simulink model "Copy_of_minimal_rcu_full"  (R2014b)
settings: Solver=ode4  SolverMode=SingleTasking  StartTime=0.0  StopTime=t_sim  FixedStep=sample_time_model  RelTol=1e-3
PreLoadFcn:
  | initModell
InitFcn:
  | initModell
undefined symbols (not defined in the file): FILTER_TAU_EXT, FIXED_FILTER_BANDWIDTH, FIXED_FILTER_BANDWIDTH_OBSERVER, iter, K_INV, KI2TAU_VEC, KS_trq, KT_trq, load_inertia, load_mass, MAX_CURRENT, MIN_SING_VALUE_M_CART, q0, rCEE_i, sample_time_model, sample_time_robot, tau_max
libraries: simulink x69, robotics x15, beasty_sfcns x7, lwr_dynamics x6, trafo3dLib x4, holgersRobLib x3, dspmtrx3 x1, dspinverses x1
(part 2 of 4)

== system Copy_of_minimal_rcu_full/Roboter+controller/controller/Cartesian Impedance Control/calculate Feedforward ==
  note: Transforming the velocity twist given at the EE in EE coodrinates to impedance point K and K coordnates
  note: get a feedforward term from
      |  the interpolator here
  note: get a switch for interpolator and
      | numerical derivation here
  TCP_T_EE : Inport
  EE_T_K : Inport  Port=2
  0_T_EE_des : Inport  Port=3
  enable Velocity feedforward : Inport  Port=4
  Constant : Constant  Value=0
  Ground : Ground
  Numerische Differentiation : Subsystem
  Product : Product  RndMeth=Zero
  Product1 : Product  Multiplication=Matrix(*)  RndMeth=Zero
  Product2 : Product  Multiplication=Matrix(*)  RndMeth=Zero
  Product3 : Product  Multiplication=Matrix(*)  RndMeth=Zero
  Reshape : Reshape  OutputDimensionality=Customize  OutputDimensions=[4,4]
  Reshape1 : Reshape  OutputDimensionality=Customize  OutputDimensions=[4,4]
  Selector : Selector  NumberOfDimensions=2  InputPortWidth=3  IndexOptions=Index vector (dialog),Index vector (dialog)  Indices=1:3,1:4  OutputSizes=1,1
  Switch : Switch  Criteria=u2 > Threshold
  Trafo3D Adjoint : Subsystem
      mask help: Adjoint matrix for a given frame.
  Trafo3D Inverse : trafo3dLib/Trafo3D Inverse
  check if  matrix  is SO(3) : MATLAB Function  TreatAsAtomicUnit=on
  check if  matrix  is SO(3)1 : MATLAB Function  TreatAsAtomicUnit=on
  prepare matrix : Subsystem
  select 3,1 : Selector  NumberOfDimensions=2  InputPortWidth=3  IndexOptions=Index vector (dialog),Index vector (dialog)  Indices=[1:3],[1:4]  OutputSizes=1,1
  select 3,4 : Selector  NumberOfDimensions=2  InputPortWidth=3  IndexOptions=Index vector (dialog),Index vector (dialog)  Indices=[1:3],[1:4]  OutputSizes=1,1
  TCP_T_k : Outport  OutDataTypeStr=double  PortDimensions=[3 4]
  0_T_K_des : Outport  Port=2  OutDataTypeStr=double  PortDimensions=[3 4]
  dxdes : Outport  Port=3  OutDataTypeStr=double  PortDimensions=[6 1]
  wires:
  select 3,4/1 -> TCP_T_k/1
  select 3,1/1 -> 0_T_K_des/1
  0_T_EE_des/1 -> prepare matrix/1(In1)
  EE_T_K/1 -> Reshape/1
  TCP_T_EE/1 -> Reshape1/1
  Trafo3D Adjoint/1(AdH) -> Product3/1
  Product3/1 -> Product/2
  Switch/1 -> Product3/2
  Numerische Differentiation/1(EE_dx) -> Switch/3
  Product/1 -> dxdes/1
  check if  matrix  is SO(3)/1(EE_T_K) -> Product1/2, Product2/2, Selector/1
  check if  matrix  is SO(3)1/1(TCP_T_EE) -> Product2/1
  Ground/1 -> Switch/1
  Constant/1 -> Switch/2
  Reshape/1 -> check if  matrix  is SO(3)/1(matrix)
  Reshape1/1 -> check if  matrix  is SO(3)1/1(matrix)
  prepare matrix/1(Out1) -> Product1/1, Numerische Differentiation/1(T_des)
  Product2/1 -> select 3,4/1
  Product1/1 -> select 3,1/1
  enable Velocity feedforward/1 -> Product/1
  Selector/1 -> Trafo3D Inverse/1
  Trafo3D Inverse/1 -> Trafo3D Adjoint/1(H)  "K_T_EE"

== system Copy_of_minimal_rcu_full/Roboter+controller/controller/Cartesian Impedance Control/check_settings ==
  In1 : Inport
  Add1 : Sum
  Bus Selector1 : BusSelector  OutputSignals=mEE,rC_EE,I_EE
  Compare To Zero : simulink/Logic and Bit Operations/Compare To Zero  relop===  OutDataTypeStr=uint8  ZeroCross=off
  Compare To Zero1 : simulink/Logic and Bit Operations/Compare To Zero  relop===  OutDataTypeStr=uint8  ZeroCross=off
  Compare To Zero2 : simulink/Logic and Bit Operations/Compare To Zero  relop=<  OutDataTypeStr=uint8  ZeroCross=off
  Compare To Zero3 : simulink/Logic and Bit Operations/Compare To Zero  relop=<  OutDataTypeStr=uint8  ZeroCross=off
  Compare To Zero4 : simulink/Logic and Bit Operations/Compare To Zero  relop=<  OutDataTypeStr=uint8  ZeroCross=off
  Compare To Zero5 : simulink/Logic and Bit Operations/Compare To Zero  relop=~=  OutDataTypeStr=uint8
  Constant1 : Constant  Value=load_mass
  Constant3 : Constant  Value=load_inertia
  Logical Operator : Logic  Operator=OR  Inputs=5  AllPortsSameDT=off  OutDataTypeStr=boolean
  Mux1 : Mux  Inputs=3
  Product : Product  RndMeth=Zero
  Selector : Selector  InputPortWidth=3  Indices=[1]
  Selector1 : Selector  InputPortWidth=3  Indices=[2]
  Selector2 : Selector  InputPortWidth=3  Indices=[3]
  Sum of Elements : Sum  Inputs=+
  Switch : Switch  Criteria=u2 ~= 0
  load_params : Outport
  wires:
  Constant1/1 -> Product/2
  Compare To Zero5/1 -> Product/1
  Product/1 -> Add1/1
  Bus Selector1/2 -> Mux1/2  "<rC_EE>"
  Bus Selector1/3 -> Switch/3, Sum of Elements/1, Selector/1, Selector1/1, Selector2/1  "<I_EE>"
  Bus Selector1/1 -> Compare To Zero/1, Add1/2, Compare To Zero5/1  "<mEE>"
  In1/1 -> Bus Selector1/1
  Mux1/1 -> load_params/1
  Compare To Zero/1 -> Logical Operator/1
  Add1/1 -> Mux1/1
  Constant3/1 -> Switch/1
  Sum of Elements/1 -> Compare To Zero1/1
  Compare To Zero1/1 -> Logical Operator/2
  Compare To Zero2/1 -> Logical Operator/3
  Compare To Zero3/1 -> Logical Operator/4
  Compare To Zero4/1 -> Logical Operator/5
  Selector/1 -> Compare To Zero2/1
  Selector1/1 -> Compare To Zero3/1
  Selector2/1 -> Compare To Zero4/1
  Logical Operator/1 -> Switch/2
  Switch/1 -> Mux1/3

== system Copy_of_minimal_rcu_full/Roboter+controller/controller/Cartesian Impedance Control/easy interpolate ==
  desire : Inport
  rate : Inport  Port=2
  Clock : Clock
  Compare To Constant : simulink/Logic and Bit Operations/Compare To Constant  relop=<=  const=0.001  OutDataTypeStr=uint8  ZeroCross=off
  Logical Operator : Logic  Operator=OR  AllPortsSameDT=off  OutDataTypeStr=boolean
  Relational Operator : RelationalOperator  Operator=~=  OutDataTypeStr=boolean
  Unit Delay : UnitDelay  SampleTime=-1
  easy interpolator inside : Subsystem
  Out : Outport
  wires:
  desire/1 -> easy interpolator inside/1(desire), Relational Operator/2
  rate/1 -> easy interpolator inside/2(rate)
  easy interpolator inside/1(Out) -> Unit Delay/1, Out/1
  Relational Operator/1 -> Logical Operator/1
  Unit Delay/1 -> Relational Operator/1
  Clock/1 -> Compare To Constant/1
  Compare To Constant/1 -> Logical Operator/2
  Logical Operator/1 -> easy interpolator inside/Enable

== system Copy_of_minimal_rcu_full/Roboter+controller/controller/Cartesian Impedance Control/make matrix ==
  In1 : Inport
  Bus Selector1 : BusSelector  OutputSignals=dynamics_q.G,dynamics_q.Mass
  Matrix Concatenation : Concatenate  NumInputs=3  Mode=Multidimensional array  ConcatenateDimension=2
  Reshape1 : Reshape  OutputDimensionality=Customize  OutputDimensions=[7,7]
  zeros : Constant  Value=zeros(7,1)  VectorParams1D=off
  Out1 : Outport
  wires:
  Reshape1/1 -> Matrix Concatenation/3
  Bus Selector1/2 -> Reshape1/1  "<Mass>"
  Bus Selector1/1 -> Matrix Concatenation/1  "<G>"
  In1/1 -> Bus Selector1/1
  Matrix Concatenation/1 -> Out1/1
  zeros/1 -> Matrix Concatenation/2

== system Copy_of_minimal_rcu_full/Roboter+controller/controller/Joint Impedance/JOINT_IMPEDANCE_CONTROL ==
  theta : Inport
  theta_d : Inport  Port=2
  dtheta_d : Inport  Port=3
  ddtheta_d : Inport  Port=4
  enable FFWD_vel : Inport  Port=5
  enable FFWD_acc : Inport  Port=6
  joint_comp_params : Inport  Port=7
  M(theta) : Inport  Port=8
  g(theta) : Inport  Port=9
  dtheta : Inport  Port=10
  B_theta : Inport  Port=11
  Enable : EnablePort
  Joint Compliance Control : Subsystem  TreatAsAtomicUnit=on
  tau_d : Outport
  wires:
  theta/1 -> Joint Compliance Control/2(theta)
  joint_comp_params/1 -> Joint Compliance Control/4(params)
  theta_d/1 -> Joint Compliance Control/1(theta_d)
  M(theta)/1 -> Joint Compliance Control/3(M(theta))
  Joint Compliance Control/1(tau_d) -> tau_d/1
  g(theta)/1 -> Joint Compliance Control/5(g(theta))
  dtheta/1 -> Joint Compliance Control/6(dtheta)
  B_theta/1 -> Joint Compliance Control/7(B_theta)
  dtheta_d/1 -> Joint Compliance Control/8(dtheta_d)
  enable FFWD_vel/1 -> Joint Compliance Control/10(enable FFWD_Vel)
  ddtheta_d/1 -> Joint Compliance Control/9(ddtheta_d)
  enable FFWD_acc/1 -> Joint Compliance Control/11(enable FFWD_Acc)

== system Copy_of_minimal_rcu_full/Roboter+controller/controller/Joint Impedance/Joint Compliance Parameters ==
  K_theta : Inport
  D_theta : Inport  Port=2
  Iterations : Constant  Value=5  OutDataTypeStr=double
  Manual Switch : ManualSwitch
  Mux1 : Mux  Inputs=5
  NO stiffness correction : Constant  Value=0  OutDataTypeStr=double
  Saturation : Saturate  UpperLimit=[2000 2000 2000 2000 2000 800 2000]  LowerLimit=0.001
  Selector : Selector  InputPortWidth=7
  WITH stiffness correction : Constant  OutDataTypeStr=double
  delay : Constant  Value=0  OutDataTypeStr=double
  interpol1 : Subsystem
  interpol2 : Subsystem
  all : Outport
  wires:
  Mux1/1 -> all/1
  NO stiffness correction/1 -> Manual Switch/1
  WITH stiffness correction/1 -> Manual Switch/2
  Iterations/1 -> Mux1/3
  Manual Switch/1 -> Mux1/4
  delay/1 -> Mux1/5
  K_theta/1 -> interpol1/1(In1)
  Saturation/1 -> Mux1/1
  D_theta/1 -> interpol2/1(In1)
  Selector/1 -> Mux1/2
  interpol1/1(Out1) -> Saturation/1
  interpol2/1(Out1) -> Selector/1

== system Copy_of_minimal_rcu_full/Roboter+controller/controller/Joint Impedance/Velocity Filter ==
  q : Inport
  Discrete Filter1 : Subsystem
  Subsystem : Subsystem
  dq : Outport
  wires:
  Discrete Filter1/1(dq_filt) -> dq/1
  q/1 -> Subsystem/1(u), Subsystem/2(y_init)
  Subsystem/1(y) -> Discrete Filter1/1(dq)

== system Copy_of_minimal_rcu_full/Roboter+controller/controller/gains_selector/K_imp ==
  KS_imp : Constant  Value=KS_trq.*[1 1 1 1 1 1 1]*1.0
  KT_imp : Constant  Value=KT_trq.*[1 1 1 1 1 1 1].*[0.8 0.8 0.7 0.8 0.8 0.8 0.8]
  Mux2 : Mux  Inputs=2
  Reshape : Reshape
  K_T : Outport
  K : Outport  Port=2
  wires:
  Mux2/1 -> Reshape/1  "K_imp"
  KS_imp/1 -> Mux2/1
  KT_imp/1 -> Mux2/2, K_T/1  "KT_imp"
  Reshape/1 -> K/1

== system Copy_of_minimal_rcu_full/Roboter+controller/controller/gains_selector/K_imp_joint ==
  KS_imp_joint : Constant  Value=KS_trq.*[1 1 1 1 1 1 1]*1.2
  KT_imp_joint : Constant  Value=KT_trq.*[1 1 1 1 1 1 1].*[1 1 1.2 1 1 1 1]
  Mux4 : Mux  Inputs=2
  Reshape : Reshape
  K_T : Outport
  K : Outport  Port=2
  wires:
  KS_imp_joint/1 -> Mux4/1
  Mux4/1 -> Reshape/1
  Reshape/1 -> K/1
  KT_imp_joint/1 -> Mux4/2, K_T/1  "KT_imp_joint"

== system Copy_of_minimal_rcu_full/Roboter+controller/robot_simulation/Dynamics/Joint Dynamic ==
  note: Calculates the elastic joints from
      | BJoint*d^2theta/dt^2 +KJoint(theta-q)+DJoint/KJoint*(dtheta/dt-dq/dt)+DvisJoint*dtheta/dt = tau_m
      |
      | STANDARD PARAMETERS
      | KJoint = [6900 10854.7 10000 10000 6464.3 10000 10000]
      | BJoint = [4.155 4.155 3.616 1.385 0.541 0.60083 0.60083]
      | DvisJoint = [20 16.98 16.6 24 18 12 12]
      | DJoint = [0 0 0 0 0 0 0]
      | TauMaxJoint = [180 180 80 80 30 30 30]
      |
      | INPUTS
      |    q joint angles
      |    dq/dt joint velocities
      |    tau_m motor torque
      |
      | OUTPUTS
      |    tau_a to the robot applied torque
      |    theta motor position
      |    dtheta/dt motor velocity
  q : Inport
  qd : Inport  Port=2
  tau_m : Inport  Port=3
  tehta_0 : Inport  Port=4
  1/ Bjoint : Gain  Gain=1./[4.155 4.155 3.616 1.385 0.541 0.60083 0.60083]'
  Display2 : Display
  DvisJoint : Gain  Gain=[20 16.98 16.6 24 18 12 12]'
  Integrator1 : Integrator  InitialCondition=zeros(7,1)
  Integrator2 : Integrator  InitialConditionSource=external  InitialCondition=[0; pi/4; 0; pi/4; 0; pi/4; 0]
  Sum : Sum  Inputs=|-+
  Sum1 : Sum  Inputs=|-+
  Sum2 : Sum  Inputs=-+-
  Sum3 : Sum  Inputs=|++
  dJoiunt/kJoint : Gain  Gain=zeros(7,1)
  kJoint : Gain  Gain=[6900 10854.7 10000 10000 6464.3 10000 10000]'
  kJoint1 : Gain  Gain=[6900 10854.7 10000 10000 6464.3 10000 10000]'
  tauMaxJoint : Saturate  UpperLimit=tau_max  LowerLimit=-tau_max
  tau_a : Outport
  theta : Outport  Port=2
  thetaD : Outport  Port=3
  wires:
  kJoint/1 -> dJoiunt/kJoint/1
  tauMaxJoint/1 -> tau_a/1, Sum2/1
  Sum3/1 -> tauMaxJoint/1
  1/ Bjoint/1 -> Integrator1/1
  DvisJoint/1 -> Sum2/3
  kJoint1/1 -> Sum3/2
  Sum1/1 -> kJoint/1
  Sum/1 -> kJoint1/1
  tau_m/1 -> Sum2/2
  Sum2/1 -> 1/ Bjoint/1
  qd/1 -> Sum1/1
  Integrator2/1 -> Display2/1, theta/1, Sum/2  "theta"
  q/1 -> Sum/1
  Integrator1/1 -> thetaD/1, DvisJoint/1, Integrator2/1, Sum1/2  "thetaD"
  dJoiunt/kJoint/1 -> Sum3/1
  tehta_0/1 -> Integrator2/2

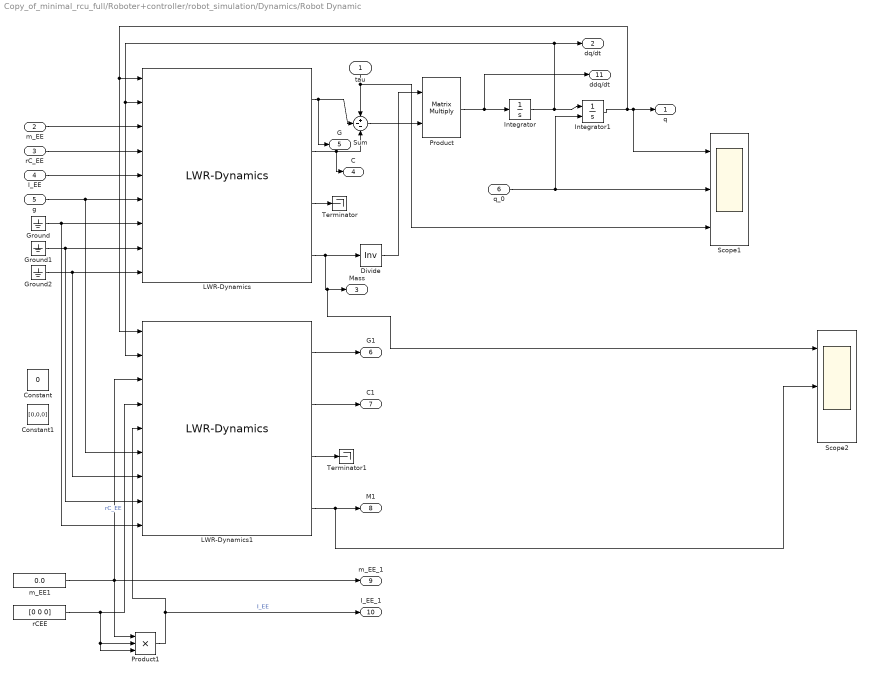
== system Copy_of_minimal_rcu_full/Roboter+controller/robot_simulation/Dynamics/Robot Dynamic ==
  tau : Inport
  m_EE : Inport  Port=2
  rC_EE : Inport  Port=3
  I_EE : Inport  Port=4
  g : Inport  Port=5
  q_0 : Inport  Port=6
  Constant : Constant  Value=0
  Constant1 : Constant  Value=[0,0,0]
  Divide : Product  Inputs=/  Multiplication=Matrix(*)
  Ground : Ground
  Ground1 : Ground
  Ground2 : Ground
  Integrator : Integrator  InitialCondition=zeros(7,1)
  Integrator1 : Integrator  InitialConditionSource=external
  LWR-Dynamics : lwr_dynamics/Dynamics/LWR-Dynamics
  LWR-Dynamics1 : lwr_dynamics/Dynamics/LWR-Dynamics
  Product : Product  Multiplication=Matrix(*)  RndMeth=Zero
  Product1 : Product  Inputs=3  RndMeth=Zero
  Scope1 : Scope  NumInputPorts=3
      settings: TimeRange=2  YMin=-2~-2~-40  YMax=1~1~20
  Scope2 : Scope  NumInputPorts=3
      settings: TimeRange=2  YMin=-0.1~-1~-0.00015  YMax=0.6~1~0.0001  SaveName=ScopeData11
  Sum : Sum  Inputs=+--
  Terminator : Terminator
  Terminator1 : Terminator
  m_EE1 : Constant  Value=0.0
  rCEE : Constant  Value=[0 0 0]
  q : Outport
  dq/dt : Outport  Port=2
  Mass : Outport  Port=3
  C : Outport  Port=4
  G : Outport  Port=5
  G1 : Outport  Port=6
  C1 : Outport  Port=7
  M1 : Outport  Port=8
  m_EE_1 : Outport  Port=9
  I_EE_1 : Outport  Port=10
  ddq/dt : Outport  Port=11
  wires:
  Integrator/1 -> Integrator1/1, dq/dt/1, LWR-Dynamics1/2, LWR-Dynamics/2
  LWR-Dynamics/4 -> Divide/1, Scope2/1, Mass/1
  LWR-Dynamics/1 -> Sum/2, G/1
  Sum/1 -> Product/2
  Integrator1/1 -> Scope1/1, q/1, LWR-Dynamics1/1, LWR-Dynamics/1
  m_EE/1 -> LWR-Dynamics/3
  rC_EE/1 -> LWR-Dynamics/4
  I_EE/1 -> LWR-Dynamics/5
  Ground/1 -> LWR-Dynamics1/9, LWR-Dynamics/7
  Ground1/1 -> LWR-Dynamics/8, LWR-Dynamics1/8
  Ground2/1 -> LWR-Dynamics/9, LWR-Dynamics1/7
  Divide/1 -> Product/1
  Product/1 -> ddq/dt/1, Integrator/1
  g/1 -> LWR-Dynamics/6, LWR-Dynamics1/6
  LWR-Dynamics/2 -> Sum/3, C/1
  tau/1 -> Sum/1, Scope1/3
  LWR-Dynamics/3 -> Terminator/1
  q_0/1 -> Integrator1/2, Scope1/2
  LWR-Dynamics1/3 -> Terminator1/1
  LWR-Dynamics1/1 -> G1/1
  LWR-Dynamics1/2 -> C1/1
  LWR-Dynamics1/4 -> Scope2/2, M1/1
  rCEE/1 -> LWR-Dynamics1/4, Product1/2, Product1/3  "rC_EE"
  m_EE1/1 -> LWR-Dynamics1/3, m_EE_1/1, Product1/1
  Product1/1 -> LWR-Dynamics1/5, I_EE_1/1  "I_EE"

== system Copy_of_minimal_rcu_full/Roboter+controller/robot_simulation/Dynamics/ZUSTANDSREGLER1 ==
  note: tau_m
  tau : Inport
  tau_d : Inport  Port=2
  Gains : Inport  Port=3
  dCG_0 : Inport  Port=4
  reset : Inport  Port=5
  CG_0 : Inport  Port=6
  Joint_controller joint_impedance : Subsystem
  Saturation : Saturate  UpperLimit=MAX_CURRENT  LowerLimit=-MAX_CURRENT
  Selctor : Selector  InputPortWidth=14  Indices=1:7
  Selctor1 : Selector  InputPortWidth=14  Indices=8:14
  Sum : Sum  Inputs=++|
  Sum1 : Sum  Inputs=|++
  Torque comp1 : Gain  Gain=KI2TAU_VEC  SaturateOnIntegerOverflow=on  OutDataTypeStr=Inherit: Same as input  ParamDataTypeStr=Inherit: Same as input
  controller cart impedance : Subsystem
  Current_des : Outport  InitialOutput=0
  wires:
  tau_d/1 -> Sum/1, Joint_controller joint_impedance/1(tau_d), controller cart impedance/1(tau_d)  "tau_d"
  Torque comp1/1 -> Saturation/1
  Saturation/1 -> Current_des/1
  CG_0/1 -> controller cart impedance/2(CG_0), Joint_controller joint_impedance/2(CG_O)  "CG_O"
  Joint_controller joint_impedance/1(I_out) -> Sum1/2
  controller cart impedance/1(I_out) -> Sum1/1
  Sum/1 -> Torque comp1/1
  reset/1 -> Joint_controller joint_impedance/5(reset), controller cart impedance/5(reset)
  Sum1/1 -> Sum/2
  Gains/1 -> Selctor/1, Selctor1/1
  dCG_0/1 -> controller cart impedance/6(dCG_0)
  tau/1 -> controller cart impedance/3(tau), Joint_controller joint_impedance/3(tau)  "tau"
  Selctor/1 -> controller cart impedance/4(Gains)
  Selctor1/1 -> Joint_controller joint_impedance/4(Gains)

== system Copy_of_minimal_rcu_full/Roboter+controller/robot_simulation/model/Body Jacobians ==
  q : Inport
  TCP_T_EE : Inport  Port=2
  Bus Creator1 : BusCreator  Inputs=8
  Jacobian LBR-M : S-Function  FunctionName=lbrmjacobitcp_sfun  EnableBusSupport=off
  Math Function : Math  Operator=transpose  SaturateOnIntegerOverflow=on
  Reshape{,1..7} (8 alike) : Reshape
  Reshape8 : Reshape  OutputDimensionality=Customize  OutputDimensions=[4,4]
  S-Function : S-Function  FunctionName=KUKA_JacobianTotTransposedSfun  Parameters=rot(1,1), rot(1,2), rot(1,3), rot(2,1), rot(2,2), rot(2,3), rot(3,1), rot(3,2), rot(3,3), tcp(1), tcp(2), tcp(3)  EnableBusSupport=off  mask{rot=eye(3), tcp=zeros(3,1)}
      mask prompts: rot "TCP-Rotation"; tcp "TCP-Translation"
  Selector : Selector  NumberOfDimensions=2  InputPortWidth=3  IndexOptions=Select all,Index vector (dialog)  Indices=-1,1:6
  Selector1 : Selector  NumberOfDimensions=2  InputPortWidth=3  IndexOptions=Select all,Index vector (dialog)  Indices=-1,7:12
  Selector2 : Selector  NumberOfDimensions=2  InputPortWidth=3  IndexOptions=Select all,Index vector (dialog)  Indices=-1,13:18
  Selector3 : Selector  NumberOfDimensions=2  InputPortWidth=3  IndexOptions=Select all,Index vector (dialog)  Indices=-1,19:24
  Selector4 : Selector  NumberOfDimensions=2  InputPortWidth=3  IndexOptions=Select all,Index vector (dialog)  Indices=-1,25:30
  Selector5 : Selector  NumberOfDimensions=2  InputPortWidth=3  IndexOptions=Select all,Index vector (dialog)  Indices=-1,31:36
  Selector6 : Selector  NumberOfDimensions=2  InputPortWidth=3  IndexOptions=Select all,Index vector (dialog)  Indices=-1,37:42
  Selector7 : Selector  NumberOfDimensions=2  InputPortWidth=3  IndexOptions=Index vector (dialog),Index vector (dialog)  Indices=1:3,1:4
  jacobians wrt body : Outport
  wires:
  Math Function/1 -> Reshape7/1
  Selector7/1 -> Jacobian LBR-M/2
  Reshape8/1 -> Selector7/1
  Reshape7/1 -> Bus Creator1/8  "B_JT_EE"
  Jacobian LBR-M/1 -> Math Function/1
  TCP_T_EE/1 -> Reshape8/1
  Bus Creator1/1 -> jacobians wrt body/1
  Reshape6/1 -> Bus Creator1/7  "B_JT_7"
  Reshape5/1 -> Bus Creator1/6  "B_JT_6"
  Reshape4/1 -> Bus Creator1/5  "B_JT_5"
  Reshape3/1 -> Bus Creator1/4  "B_JT_4"
  Reshape2/1 -> Bus Creator1/3  "B_JT_3"
  Reshape1/1 -> Bus Creator1/2  "B_JT_2"
  Reshape/1 -> Bus Creator1/1  "B_JT_1"
  q/1 -> Jacobian LBR-M/1, S-Function/1
  Selector/1 -> Reshape/1
  Selector1/1 -> Reshape1/1
  Selector2/1 -> Reshape2/1
  Selector3/1 -> Reshape3/1
  Selector4/1 -> Reshape4/1
  Selector5/1 -> Reshape5/1
  Selector6/1 -> Reshape6/1
  S-Function/1 -> Selector/1, Selector1/1, Selector2/1, Selector3/1, Selector4/1, Selector6/1, Selector5/1

== system Copy_of_minimal_rcu_full/Roboter+controller/robot_simulation/model/Jacobians to Zero ==
  q : Inport
  TCP_T_EE : Inport  Port=2
  Bus Creator1 : BusCreator  Inputs=8
  LWR Jacobian EE : lwr_dynamics/Kinematics/LWR Jacobian EE
  LWR-Jacobians : lwr_dynamics/Kinematics/LWR-Jacobians
  Reshape{1..8} (8 alike) : Reshape
  Reshape9 : Reshape  OutputDimensionality=Customize  OutputDimensions=[4,4]
  jacobians_wrt_zero : Outport
  wires:
  Reshape9/1 -> LWR Jacobian EE/2
  Reshape8/1 -> Bus Creator1/8  "O_JT_EE"
  Reshape7/1 -> Bus Creator1/7  "O_JT_7"
  Reshape6/1 -> Bus Creator1/6  "O_JT_6"
  Reshape5/1 -> Bus Creator1/5  "O_JT_5"
  Reshape3/1 -> Bus Creator1/4  "O_JT_4"
  Reshape2/1 -> Bus Creator1/3  "O_JT_3"
  Reshape1/1 -> Bus Creator1/2  "O_JT_2"
  Reshape4/1 -> Bus Creator1/1  "O_JT_1"
  q/1 -> LWR-Jacobians/1, LWR Jacobian EE/1
  LWR Jacobian EE/1 -> Reshape8/1
  LWR-Jacobians/7 -> Reshape7/1
  LWR-Jacobians/6 -> Reshape6/1
  LWR-Jacobians/5 -> Reshape5/1
  LWR-Jacobians/4 -> Reshape3/1
  LWR-Jacobians/3 -> Reshape2/1
  LWR-Jacobians/2 -> Reshape1/1
  LWR-Jacobians/1 -> Reshape4/1
  TCP_T_EE/1 -> Reshape9/1
  Bus Creator1/1 -> jacobians_wrt_zero/1

== system Copy_of_minimal_rcu_full/Roboter+controller/robot_simulation/model/forward_kin_q ==
  q : Inport
  TCP_T_EE : Inport  Port=2
  Bus Creator2 : BusCreator  Inputs=9
  Gain : Gain
  LWR-Transformations : lwr_dynamics/Kinematics/LWR-Transformations
  fkin_q : Outport
  wires:
  LWR-Transformations/8 -> Bus Creator2/9  "O_T_EE"
  Bus Creator2/1 -> fkin_q/1
  Gain/1 -> Bus Creator2/8  "O_T_TCP"
  LWR-Transformations/7 -> Bus Creator2/7, Gain/1  "O_T_7"
  LWR-Transformations/6 -> Bus Creator2/6  "O_T_6"
  LWR-Transformations/5 -> Bus Creator2/5  "O_T_5"
  LWR-Transformations/4 -> Bus Creator2/4  "O_T_4"
  LWR-Transformations/3 -> Bus Creator2/3  "O_T_3"
  LWR-Transformations/2 -> Bus Creator2/2  "O_T_2"
  LWR-Transformations/1 -> Bus Creator2/1  "O_T_1"
  q/1 -> LWR-Transformations/1
  TCP_T_EE/1 -> LWR-Transformations/2

== system Copy_of_minimal_rcu_full/Roboter+controller/robot_simulation/model/forward_kin_q1 ==
  q : Inport
  TCP_T_EE : Inport  Port=2
  Bus Creator2 : BusCreator  Inputs=9
  Gain : Gain
  LWR-Transformations : lwr_dynamics/Kinematics/LWR-Transformations
  fkin_q : Outport
  wires:
  TCP_T_EE/1 -> LWR-Transformations/2
  q/1 -> LWR-Transformations/1
  LWR-Transformations/1 -> Bus Creator2/1  "O_T_1"
  LWR-Transformations/2 -> Bus Creator2/2  "O_T_2"
  LWR-Transformations/3 -> Bus Creator2/3  "O_T_3"
  LWR-Transformations/4 -> Bus Creator2/4  "O_T_4"
  LWR-Transformations/5 -> Bus Creator2/5  "O_T_5"
  LWR-Transformations/6 -> Bus Creator2/6  "O_T_6"
  LWR-Transformations/7 -> Gain/1, Bus Creator2/7  "O_T_7"
  Gain/1 -> Bus Creator2/8  "O_T_TCP"
  Bus Creator2/1 -> fkin_q/1
  LWR-Transformations/8 -> Bus Creator2/9  "O_T_EE"

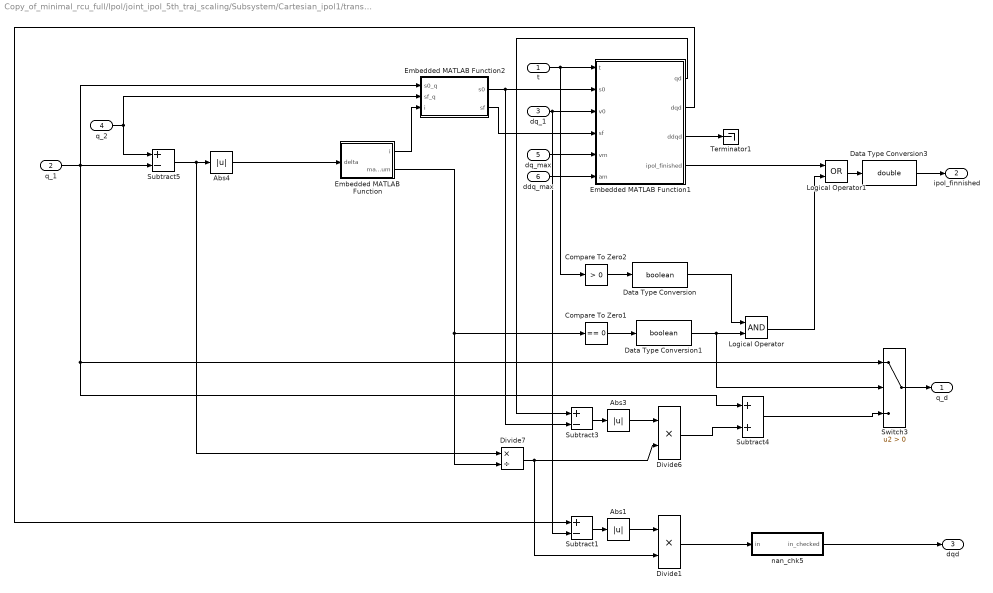
== system Copy_of_minimal_rcu_full/Ipol/joint_ipol_5th_traj_scaling/Subsystem/Cartesian_ipol1/translation ==
  t : Inport
  q_1 : Inport  Port=2
  dq_1 : Inport  Port=3
  q_2 : Inport  Port=4
  dq_max : Inport  Port=5
  ddq_max : Inport  Port=6
  Abs1 : Abs
  Abs3 : Abs
  Abs4 : Abs
  Compare To Zero1 : simulink/Logic and Bit Operations/Compare To Zero  relop===  OutDataTypeStr=uint8  ZeroCross=off
  Compare To Zero2 : simulink/Logic and Bit Operations/Compare To Zero  relop=>  OutDataTypeStr=uint8  ZeroCross=off
  Data Type Conversion : DataTypeConversion  OutDataTypeStr=boolean
  Data Type Conversion1 : DataTypeConversion  OutDataTypeStr=boolean
  Data Type Conversion3 : DataTypeConversion  OutDataTypeStr=double
  Divide1 : Product  Inputs=**
  Divide6 : Product  Inputs=**
  Divide7 : Product  Inputs=*/
  Embedded MATLAB Function : MATLAB Function  TreatAsAtomicUnit=on
  Embedded MATLAB Function1 : MATLAB Function  TreatAsAtomicUnit=on
  Embedded MATLAB Function2 : MATLAB Function  TreatAsAtomicUnit=on
  Logical Operator : Logic  AllPortsSameDT=off  OutDataTypeStr=boolean
  Logical Operator1 : Logic  Operator=OR  AllPortsSameDT=off  OutDataTypeStr=boolean
  Subtract1 : Sum  Inputs=+-
  Subtract3 : Sum  Inputs=+-
  Subtract4 : Sum
  Subtract5 : Sum  Inputs=+-
  Switch3 : Switch  Criteria=u2 > Threshold
  Terminator1 : Terminator
  nan_chk5 : Subsystem
  q_d : Outport
  ipol_finnished : Outport  Port=2
  dqd : Outport  Port=3
  wires:
  nan_chk5/1(in_checked) -> dqd/1
  Divide1/1 -> nan_chk5/1(in)
  Embedded MATLAB Function1/2(dqd) -> Subtract1/1
  Subtract1/1 -> Abs1/1
  Abs1/1 -> Divide1/1
  Divide6/1 -> Subtract4/2
  Divide7/1 -> Divide1/2, Divide6/2
  Abs4/1 -> Embedded MATLAB Function/1(delta)
  Subtract5/1 -> Divide7/1, Abs4/1
  q_1/1 -> Switch3/1, Subtract4/1, Subtract5/2, Embedded MATLAB Function2/1(s0_q)
  q_2/1 -> Subtract5/1, Embedded MATLAB Function2/2(sf_q)
  Embedded MATLAB Function/2(maximum) -> Compare To Zero1/1, Divide7/2
  Embedded MATLAB Function/1(i) -> Embedded MATLAB Function2/3(i)
  Subtract3/1 -> Abs3/1
  dq_1/1 -> Subtract1/2, Embedded MATLAB Function1/3(v0)
  dq_max/1 -> Embedded MATLAB Function1/5(vm)
  ddq_max/1 -> Embedded MATLAB Function1/6(am)
  t/1 -> Embedded MATLAB Function1/1(t), Compare To Zero2/1
  Embedded MATLAB Function2/1(s0) -> Embedded MATLAB Function1/2(s0), Subtract3/2
  Embedded MATLAB Function2/2(sf) -> Embedded MATLAB Function1/4(sf)
  Embedded MATLAB Function1/1(qd) -> Subtract3/1
  Embedded MATLAB Function1/3(ddqd) -> Terminator1/1
  Abs3/1 -> Divide6/1
  Logical Operator/1 -> Logical Operator1/2
  Data Type Conversion/1 -> Logical Operator/1
  Data Type Conversion1/1 -> Logical Operator/2, Switch3/2
  Compare To Zero1/1 -> Data Type Conversion1/1
  Embedded MATLAB Function1/4(ipol_finished) -> Logical Operator1/1
  Logical Operator1/1 -> Data Type Conversion3/1
  Data Type Conversion3/1 -> ipol_finnished/1
  Subtract4/1 -> Switch3/3
  Switch3/1 -> q_d/1
  Compare To Zero2/1 -> Data Type Conversion/1

== system Copy_of_minimal_rcu_full/Ipol/joint_ipol_5th_traj_scaling/Subsystem/time_generator and resets/Triggered Subsystem ==
  t : Inport
  Trigger : TriggerPort
  t0 : Outport
  wires:
  t/1 -> t0/1

== system Copy_of_minimal_rcu_full/Roboter+controller/State_Observer/Impulse_Observer/Subsystem1/calc_beta ==
  M : Inport
  dq : Inport  Port=2
  n : Inport  Port=3
  Discrete Derivative : simulink/Discrete/Discrete Derivative  gainval=1.0  ICPrevScaledInput=0.0  InputProcessing=Inherited  OutMin=[]  OutMax=[]  OutDataType=sfix(16)  OutScaling=2^-10  DoSatur=off
  Product : Product  Multiplication=Matrix(*)  RndMeth=Zero
  Reshape1 : Reshape  OutputDimensionality=Column vector (2-D)
  Reshape2 : Reshape
  Sum6 : Sum  Inputs=+-
  "beta " : Outport
  dM : Outport  Port=2
  dMdq2 : Outport  Port=3
  wires:
  Product/1 -> Reshape2/1
  Discrete Derivative/1 -> dM/1, Product/1
  Sum6/1 -> "beta "/1
  n/1 -> Sum6/1
  M/1 -> Discrete Derivative/1
  dq/1 -> Reshape1/1
  Reshape1/1 -> Product/2
  Reshape2/1 -> dMdq2/1, Sum6/2

== system Copy_of_minimal_rcu_full/Roboter+controller/State_Observer/Impulse_Observer/Subsystem1/calc_p ==
  M : Inport
  dq : Inport  Port=2
  Product : Product  Multiplication=Matrix(*)  RndMeth=Zero
  Reshape : Reshape  OutputDimensionality=Column vector (2-D)
  p : Outport
  wires:
  dq/1 -> Reshape/1
  M/1 -> Product/1
  Product/1 -> p/1
  Reshape/1 -> Product/2

== system Copy_of_minimal_rcu_full/Roboter+controller/controller/Cartesian Impedance Control/Cartesian Compliance Parameters1/damping type ==
  Controller type : Constant  Value=damping_type  OutDataTypeStr=double
  Out1 : Outport
  wires:
  Controller type/1 -> Out1/1

== system Copy_of_minimal_rcu_full/Roboter+controller/controller/Cartesian Impedance Control/Cartesian Compliance Parameters1/interpol ==
  In1 : Inport
  Easy Ipol_MIMO : beasty_sfcns/Utility Functions/Easy Ipol_MIMO  h=sample_time_robot  n=6
  K rates : Constant  Value=[2000 2000 2000 600 600 600]
  Out1 : Outport
  wires:
  In1/1 -> Easy Ipol_MIMO/1
  Easy Ipol_MIMO/1 -> Out1/1  "K_x"
  K rates/1 -> Easy Ipol_MIMO/2, Easy Ipol_MIMO/3

== system Copy_of_minimal_rcu_full/Roboter+controller/controller/Cartesian Impedance Control/Cartesian Compliance Parameters1/interpol5 ==
  In1 : Inport
  Easy Ipol_MIMO : beasty_sfcns/Utility Functions/Easy Ipol_MIMO  h=sample_time_robot  n=6
  K rates3 : Constant  Value=[1 1 1 1 1 1]
  Out1 : Outport
  wires:
  K rates3/1 -> Easy Ipol_MIMO/2, Easy Ipol_MIMO/3
  In1/1 -> Easy Ipol_MIMO/1
  Easy Ipol_MIMO/1 -> Out1/1

== system Copy_of_minimal_rcu_full/Roboter+controller/controller/Cartesian Impedance Control/Cartesian Compliance Parameters1/stiffness type ==
  Controller type : Constant  Value=controller_type  OutDataTypeStr=double
  Out1 : Outport
  wires:
  Controller type/1 -> Out1/1

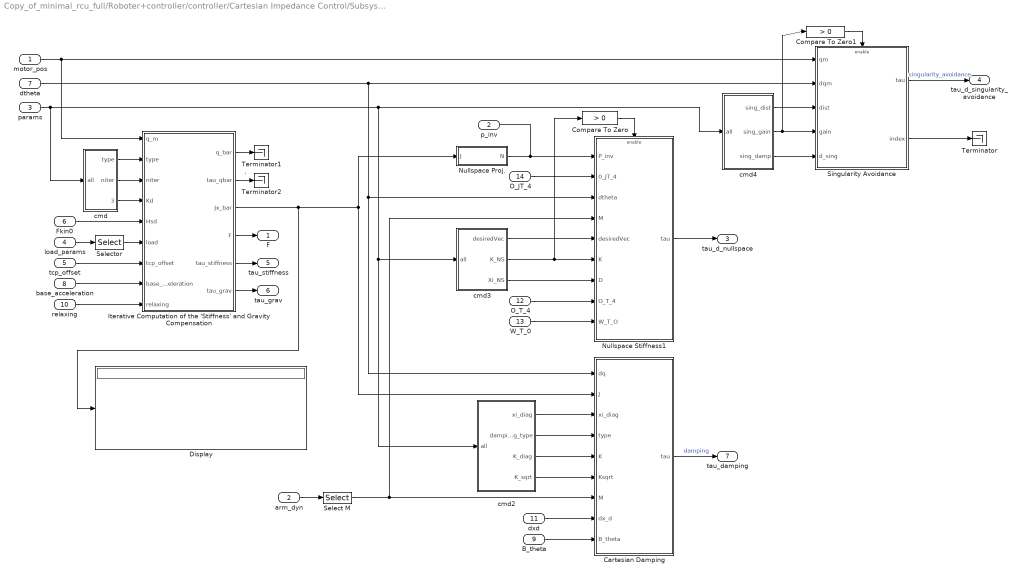
== system Copy_of_minimal_rcu_full/Roboter+controller/controller/Cartesian Impedance Control/Subsystem/Cartesian Compliance Control ==
  motor_pos : Inport
  arm_dyn : Inport  Port=2
  params : Inport  Port=3
  load_params : Inport  Port=4
  tcp_offset : Inport  Port=5
  Fkin0 : Inport  Port=6
  dtheta : Inport  Port=7
  base_acceleration : Inport  Port=8
  B_theta : Inport  Port=9
  relaxing : Inport  Port=10
  dxd : Inport  Port=11
  O_T_4 : Inport  Port=12
  W_T_0 : Inport  Port=13
  O_JT_4 : Inport  Port=14
  Cartesian Damping : Subsystem  TreatAsAtomicUnit=on
  Compare To Zero : simulink/Logic and Bit Operations/Compare To Zero  relop=>  OutDataTypeStr=uint8  ZeroCross=off
  Compare To Zero1 : simulink/Logic and Bit Operations/Compare To Zero  relop=>  OutDataTypeStr=uint8  ZeroCross=off
  Display : Display
  Iterative Computation of the 'Stiffness' and Gravity Compensation : Subsystem  TreatAsAtomicUnit=on
  Nullspace Proj. : MATLAB Function  TreatAsAtomicUnit=on
  Nullspace Stiffness1 : Subsystem  TreatAsAtomicUnit=on
  Select M : Selector  NumberOfDimensions=2  InputPortWidth=3  IndexOptions=Select all,Index vector (dialog)  Indices=-1,3:9
  Selector : Selector  InputPortWidth=7  Indices=1:4
  Singularity Avoidance : Subsystem  TreatAsAtomicUnit=on
  Terminator : Terminator
  Terminator1 : Terminator
  Terminator2 : Terminator
  cmd : Subsystem
  cmd2 : Subsystem
  cmd3 : Subsystem
  cmd4 : Subsystem
  F : Outport  OutDataTypeStr=double  PortDimensions=6
  p_inv : Outport  Port=2  OutDataTypeStr=double  PortDimensions=[7 7]
  tau_d_nullspace : Outport  Port=3  OutDataTypeStr=double  PortDimensions=7
  tau_d_singularity_avoidance : Outport  Port=4  OutDataTypeStr=double  PortDimensions=7
  tau_stiffness : Outport  Port=5  OutDataTypeStr=double  PortDimensions=7
  tau_grav : Outport  Port=6  OutDataTypeStr=double  PortDimensions=7
  tau_damping : Outport  Port=7  OutDataTypeStr=double  PortDimensions=7
  wires:
  base_acceleration/1 -> Iterative Computation of the 'Stiffness' and Gravity Compensation/8(base_acceleration)
  load_params/1 -> Selector/1
  arm_dyn/1 -> Select M/1
  params/1 -> cmd/1(all), cmd2/1(all), cmd3/1(all), cmd4/1(all)
  Singularity Avoidance/1(tau) -> tau_d_singularity_avoidance/1  "singularity_avoidance"
  Compare To Zero/1 -> Nullspace Stiffness1/Enable
  Compare To Zero1/1 -> Singularity Avoidance/Enable
  Cartesian Damping/1(tau) -> tau_damping/1  "damping"
  cmd/3(K_diag) -> Iterative Computation of the 'Stiffness' and Gravity Compensation/4(Kd)
  Iterative Computation of the 'Stiffness' and Gravity Compensation/3(Jx_bar) -> Display/1, Nullspace Proj./1(J), Cartesian Damping/2(J)
  cmd/2(niter) -> Iterative Computation of the 'Stiffness' and Gravity Compensation/3(niter)
  Selector/1 -> Iterative Computation of the 'Stiffness' and Gravity Compensation/6(load)
  cmd/1(type) -> Iterative Computation of the 'Stiffness' and Gravity Compensation/2(type)
  Fkin0/1 -> Iterative Computation of the 'Stiffness' and Gravity Compensation/5(Hsd)
  Iterative Computation of the 'Stiffness' and Gravity Compensation/4(F) -> F/1
  tcp_offset/1 -> Iterative Computation of the 'Stiffness' and Gravity Compensation/7(tcp_offset)
  motor_pos/1 -> Singularity Avoidance/1(qm), Iterative Computation of the 'Stiffness' and Gravity Compensation/1(q_m)
  B_theta/1 -> Cartesian Damping/9(B_theta)
  relaxing/1 -> Iterative Computation of the 'Stiffness' and Gravity Compensation/9(relaxing)
  dxd/1 -> Cartesian Damping/8(dx_d)
  Nullspace Stiffness1/1(tau) -> tau_d_nullspace/1
  O_T_4/1 -> Nullspace Stiffness1/8(O_T_4)
  W_T_0/1 -> Nullspace Stiffness1/9(W_T_O)
  Nullspace Proj./1(N) -> Nullspace Stiffness1/1(P_inv), p_inv/1
  Iterative Computation of the 'Stiffness' and Gravity Compensation/1(q_bar) -> Terminator1/1
  Iterative Computation of the 'Stiffness' and Gravity Compensation/2(tau_qbar) -> Terminator2/1  "'"
  Singularity Avoidance/2(index) -> Terminator/1
  O_JT_4/1 -> Nullspace Stiffness1/2(0_JT_4)
  Select M/1 -> Cartesian Damping/7(M), Nullspace Stiffness1/4(M)
  Iterative Computation of the 'Stiffness' and Gravity Compensation/5(tau_stiffness) -> tau_stiffness/1
  Iterative Computation of the 'Stiffness' and Gravity Compensation/6(tau_grav) -> tau_grav/1
  cmd2/1(xi_diag) -> Cartesian Damping/3(xi_diag)
  cmd2/2(damping_type) -> Cartesian Damping/4(type)
  cmd2/3(K_diag) -> Cartesian Damping/5(K)
  cmd2/4(K_sqrt) -> Cartesian Damping/6(Ksqrt)
  dtheta/1 -> Cartesian Damping/1(dq), Nullspace Stiffness1/3(dtheta), Singularity Avoidance/2(dqm)
  cmd3/1(desiredVec) -> Nullspace Stiffness1/5(desiredVec)
  cmd3/2(K_NS) -> Nullspace Stiffness1/6(K), Compare To Zero/1
  cmd3/3(Xi_NS) -> Nullspace Stiffness1/7(D)
  cmd4/1(sing_dist) -> Singularity Avoidance/3(dist)
  cmd4/2(sing_gain) -> Singularity Avoidance/4(gain), Compare To Zero1/1
  cmd4/3(sing_damp) -> Singularity Avoidance/5(d_sing)

== system Copy_of_minimal_rcu_full/Roboter+controller/controller/Cartesian Impedance Control/Velocity Filter/Discrete Filter1 ==
  dq : Inport
  Add1 : Sum
  Gain1 : Gain  Gain=1/10
  Gain2 : Gain  Gain=9/10
  Unit Delay : UnitDelay  SampleTime=-1
  dq_filt : Outport  OutDataTypeStr=double  PortDimensions=7
  wires:
  dq/1 -> Gain1/1
  Gain1/1 -> Add1/1
  Gain2/1 -> Add1/2
  Add1/1 -> dq_filt/1, Unit Delay/1
  Unit Delay/1 -> Gain2/1

== system Copy_of_minimal_rcu_full/Roboter+controller/controller/Cartesian Impedance Control/calculate Feedforward/Numerische Differentiation ==
  note: Rotate the velocities 0_dx at EE from base coordinates 0 in EE coordinates
  T_des : Inport
  Product2 : Product  Multiplication=Matrix(*)  RndMeth=Zero
  Rotate_wrench1 : Subsystem
      mask help: Adjoint matrix for a given frame.
  Selector : Selector  NumberOfDimensions=2  InputPortWidth=3  IndexOptions=Index vector (dialog),Index vector (dialog)  Indices=1:3,1:4  OutputSizes=1,1
  Trafo3D Inverse : trafo3dLib/Trafo3D Inverse
  nan_chk4 : Subsystem
  numerical differentiation : Subsystem
  EE_dx : Outport
  wires:
  Rotate_wrench1/1(A_R_B) -> nan_chk4/1(in)
  numerical differentiation/1(0_dx) -> Product2/2  "0_dx"
  nan_chk4/1(in_checked) -> Product2/1
  T_des/1 -> numerical differentiation/1(T_des), Selector/1
  Product2/1 -> EE_dx/1
  Trafo3D Inverse/1 -> Rotate_wrench1/1(A_T_B)
  Selector/1 -> Trafo3D Inverse/1

== system Copy_of_minimal_rcu_full/Roboter+controller/controller/Cartesian Impedance Control/calculate Feedforward/Trafo3D Adjoint ==
  H : Inport
  0 : Constant  Value=zeros(3,3)  VectorParams1D=off
  Cross-Product : trafo3dLib/Cross-Product  SystemSampleTime=-1
  Matrix Concatenation : Concatenate  Mode=Multidimensional array  ConcatenateDimension=2
  Matrix Concatenation1 : Concatenate  Mode=Multidimensional array
  Matrix Concatenation2 : Concatenate  Mode=Multidimensional array  ConcatenateDimension=2
  R : Selector  NumberOfDimensions=2  InputPortWidth=3  IndexOptions=Index vector (dialog),Index vector (dialog)  Indices=[1,2,3],[1 2 3]
  p : Selector  NumberOfDimensions=2  InputPortWidth=3  IndexOptions=Index vector (dialog),Index vector (dialog)  Indices=[1 2 3],4
  AdH : Outport
  wires:
  Matrix Concatenation1/1 -> AdH/1
  Matrix Concatenation2/1 -> Matrix Concatenation1/2
  Cross-Product/1 -> Matrix Concatenation/2
  Matrix Concatenation/1 -> Matrix Concatenation1/1
  0/1 -> Matrix Concatenation2/1
  H/1 -> p/1, R/1
  p/1 -> Cross-Product/1
  R/1 -> Cross-Product/2, Matrix Concatenation2/2, Matrix Concatenation/1

== system Copy_of_minimal_rcu_full/Roboter+controller/controller/Cartesian Impedance Control/calculate Feedforward/prepare matrix ==
  In1 : Inport
  Constant1 : Constant  Value=[0 0 0 1]  VectorParams1D=off
  Matrix Concatenate : Concatenate  Mode=Multidimensional array
  Reshape2 : Reshape  OutputDimensionality=Customize  OutputDimensions=[3,4]
  Out1 : Outport
  wires:
  Reshape2/1 -> Matrix Concatenate/1
  Constant1/1 -> Matrix Concatenate/2
  Matrix Concatenate/1 -> Out1/1
  In1/1 -> Reshape2/1

== system Copy_of_minimal_rcu_full/Roboter+controller/controller/Cartesian Impedance Control/easy interpolate/easy interpolator inside ==
  desire : Inport
  rate : Inport  Port=2
  Enable : EnablePort
  Abs : Abs
  Detect Change : simulink/Logic and Bit Operations/Detect Change  vinit=0  InputProcessing=Inherited  OutDataTypeStr=uint8
  Discrete-Time Integrator : DiscreteIntegrator  ExternalReset=rising  InitialConditionSource=external  SampleTime=-1
  Display{1..7} (7 alike) : Display
  MinMax : MinMax  Inputs=2
  MinMax1 : MinMax  Function=max  Inputs=2
  Product : Product  RndMeth=Zero
  Saturation Dynamic : simulink/Discontinuities/Saturation Dynamic  OutMin=[]  OutMax=[]  OutDataTypeStr=Inherit: Same as second input  OutDataType=sfix(16)  OutScaling=2^-10  DoSatur=off
  Unit Delay External IC : simulink/Additional Math & Discrete/Additional Discrete/Unit Delay External IC  tsamp=-1
  correct sign : Subsystem
  memorize last : Subsystem
  Out : Outport
  wires:
  desire/1 -> memorize last/1(In1), correct sign/2(In2), Detect Change/1, MinMax1/1, MinMax/1, Unit Delay External IC/2, Display2/1
  memorize last/1(Out1) -> correct sign/1(In1), MinMax1/2, MinMax/2, Display7/1
  rate/1 -> Abs/1
  correct sign/1(Out1) -> Product/1
  Abs/1 -> Product/2
  Product/1 -> Discrete-Time Integrator/1
  Detect Change/1 -> Discrete-Time Integrator/2
  Discrete-Time Integrator/1 -> Saturation Dynamic/2, Display4/1
  MinMax1/1 -> Display1/1, Saturation Dynamic/1, Display5/1
  MinMax/1 -> Saturation Dynamic/3, Display6/1
  Saturation Dynamic/1 -> Out/1, Unit Delay External IC/1, Display3/1
  Unit Delay External IC/1 -> Discrete-Time Integrator/3

== system Copy_of_minimal_rcu_full/Roboter+controller/controller/Joint Impedance/JOINT_IMPEDANCE_CONTROL/Joint Compliance Control ==
  theta_d : Inport
  theta : Inport  Port=2
  M(theta) : Inport  Port=3
  params : Inport  Port=4
  g(theta) : Inport  Port=5
  dtheta : Inport  Port=6
  B_theta : Inport  Port=7
  dtheta_d : Inport  Port=8
  ddtheta_d : Inport  Port=9
  enable FFWD_Vel : Inport  Port=10
  enable FFWD_Acc : Inport  Port=11
  Add : Sum
  Damping Design via Generalized Eigenvalues : Subsystem
  Embedded MATLAB Function : MATLAB Function  TreatAsAtomicUnit=on
  Multiport Switch1 : MultiPortSwitch  DataPortOrder=Zero-based contiguous  Inputs=6  zeroidx=on
  NAN_checks : Subsystem
  Pragmatic Solution : Subsystem  TreatAsAtomicUnit=on
  Reshape1 : Reshape  OutputDimensionality=Customize  OutputDimensions=[7,7]
  Unit Delay{,1..4} (5 alike) : UnitDelay  SampleTime=sample_time_model
  cmd : Subsystem
  tau_d : Outport
  wires:
  params/1 -> cmd/1(all)
  cmd/1(K_diag) -> Embedded MATLAB Function/1(u), Pragmatic Solution/6(K_diag), NAN_checks/5(K_diag)
  Embedded MATLAB Function/1(y) -> Damping Design via Generalized Eigenvalues/2(K)
  M(theta)/1 -> Reshape1/1
  dtheta/1 -> Pragmatic Solution/4(dqm), NAN_checks/3(dqm)
  cmd/2(xi_diag) -> Damping Design via Generalized Eigenvalues/3(damp_fac)
  cmd/4(stiffness_correction) -> Pragmatic Solution/7(stiffness correction), NAN_checks/6(stiffness correction)
  Add/1 -> Damping Design via Generalized Eigenvalues/1(M), Pragmatic Solution/1(M)
  Unit Delay/1 -> Unit Delay1/1, Multiport Switch1/3
  Unit Delay1/1 -> Unit Delay2/1, Multiport Switch1/4
  Unit Delay2/1 -> Unit Delay3/1, Multiport Switch1/5
  theta/1 -> Multiport Switch1/2, Unit Delay/1
  Unit Delay3/1 -> Multiport Switch1/6, Unit Delay4/1
  Unit Delay4/1 -> Multiport Switch1/7
  Multiport Switch1/1 -> Pragmatic Solution/3(qm), NAN_checks/2(qm)
  cmd/3(delay) -> Multiport Switch1/1
  theta_d/1 -> Pragmatic Solution/5(qm_d), NAN_checks/4(qm_d)
  g(theta)/1 -> Pragmatic Solution/8(g(theta)), NAN_checks/7(g(theta))
  Reshape1/1 -> Add/1
  B_theta/1 -> Add/2
  dtheta_d/1 -> Pragmatic Solution/9(dqm_d)
  enable FFWD_Vel/1 -> Pragmatic Solution/10(enable FFWD vel)
  Damping Design via Generalized Eigenvalues/1(D) -> Pragmatic Solution/2(D), NAN_checks/1(D)
  Pragmatic Solution/1(tau_d) -> tau_d/1, NAN_checks/8(tau)
  ddtheta_d/1 -> Pragmatic Solution/11(ddqm_d)
  enable FFWD_Acc/1 -> Pragmatic Solution/12(enable FFWD acc)

== system Copy_of_minimal_rcu_full/Roboter+controller/controller/Joint Impedance/Joint Compliance Parameters/interpol1 ==
  In1 : Inport
  Easy Ipol_MIMO : beasty_sfcns/Utility Functions/Easy Ipol_MIMO  h=sample_time_robot  n=7
  K rates1 : Constant  Value=[2000 2000 2000 2000 2000 2000 2000]*0.05
  Out1 : Outport
  wires:
  K rates1/1 -> Easy Ipol_MIMO/3, Easy Ipol_MIMO/2
  In1/1 -> Easy Ipol_MIMO/1
  Easy Ipol_MIMO/1 -> Out1/1

== system Copy_of_minimal_rcu_full/Roboter+controller/controller/Joint Impedance/Joint Compliance Parameters/interpol2 ==
  In1 : Inport
  Easy Ipol_MIMO : beasty_sfcns/Utility Functions/Easy Ipol_MIMO  h=sample_time_robot  n=7
  K rates1 : Constant  Value=[2000 2000 2000 2000 2000 2000 2000]
  Out1 : Outport
  wires:
  K rates1/1 -> Easy Ipol_MIMO/2, Easy Ipol_MIMO/3
  In1/1 -> Easy Ipol_MIMO/1
  Easy Ipol_MIMO/1 -> Out1/1

== system Copy_of_minimal_rcu_full/Roboter+controller/controller/Joint Impedance/Velocity Filter/Discrete Filter1 ==
  dq : Inport
  Add1 : Sum
  Gain1 : Gain  Gain=1/10
  Gain2 : Gain  Gain=9/10
  Unit Delay : UnitDelay  SampleTime=-1
  dq_filt : Outport
  wires:
  Unit Delay/1 -> Gain2/1
  Add1/1 -> Unit Delay/1, dq_filt/1
  Gain2/1 -> Add1/2
  Gain1/1 -> Add1/1
  dq/1 -> Gain1/1

== system Copy_of_minimal_rcu_full/Roboter+controller/controller/Joint Impedance/Velocity Filter/Subsystem ==
  u : Inport
  y_init : Inport  Port=2
  Sum : Sum  Inputs=|+-
  Unit Delay External IC : simulink/Additional Math & Discrete/Additional Discrete/Unit Delay External IC  tsamp=-1
  Weighted Sample Time Math : Subsystem
  y : Outport
  wires:
  y_init/1 -> Unit Delay External IC/2
  u/1 -> Unit Delay External IC/1, Sum/1
  Unit Delay External IC/1 -> Sum/2
  Sum/1 -> y/1

== system Copy_of_minimal_rcu_full/Roboter+controller/robot_simulation/Dynamics/ZUSTANDSREGLER1/Joint_controller joint_impedance ==
  tau_d : Inport
  CG_O : Inport  Port=2
  tau : Inport  Port=3
  Gains : Inport  Port=4
  reset : Inport  Port=5
  First_order_filter_MIMO : beasty_sfcns/Utility Functions/First_order_filter_MIMO  h=sample_time_robot  T=1./(2*pi*FIXED_FILTER_BANDWIDTH)  nr=7
  Product : Product  SaturateOnIntegerOverflow=on  InputSameDT=on  OutDataTypeStr=Inherit: Same as first input
  Sum4 : Sum  Inputs=+-  SaturateOnIntegerOverflow=on  InputSameDT=on  OutDataTypeStr=Inherit: Same as first input
  I_out : Outport
  wires:
  Sum4/1 -> First_order_filter_MIMO/1
  First_order_filter_MIMO/1 -> Product/2
  tau_d/1 -> Sum4/1
  tau/1 -> Sum4/2
  CG_O/1 -> First_order_filter_MIMO/2
  reset/1 -> First_order_filter_MIMO/3
  Gains/1 -> Product/1
  Product/1 -> I_out/1

== system Copy_of_minimal_rcu_full/Roboter+controller/robot_simulation/Dynamics/ZUSTANDSREGLER1/controller cart impedance ==
  tau_d : Inport
  CG_0 : Inport  Port=2
  tau : Inport  Port=3
  Gains : Inport  Port=4
  reset : Inport  Port=5
  dCG_0 : Inport  Port=6
  First_order_filter_MIMO1 : beasty_sfcns/Utility Functions/First_order_filter_MIMO  h=sample_time_robot  T=1./(2*pi*FIXED_FILTER_BANDWIDTH)  nr=7
  Product1 : Product  SaturateOnIntegerOverflow=on  InputSameDT=on  OutDataTypeStr=Inherit: Same as first input
  Reshape1 : Reshape
  Sum3 : Sum  Inputs=+-  SaturateOnIntegerOverflow=on  InputSameDT=on  OutDataTypeStr=Inherit: Same as first input
  num. derivative : Subsystem  TreatAsAtomicUnit=on  mask{h=sample_time_model}
      mask help:
      | discrete derivative for vector inputs
      | h - sampling time
  num. derivative2 : Subsystem  TreatAsAtomicUnit=on  mask{h=sample_time_model}
      mask help:
      | discrete derivative for vector inputs
      | h - sampling time
  I_out : Outport
  wires:
  num. derivative/1(y[n]) -> Sum3/1
  num. derivative2/1(y[n]) -> Sum3/2
  Sum3/1 -> First_order_filter_MIMO1/1
  First_order_filter_MIMO1/1 -> Product1/2
  Gains/1 -> Product1/1
  dCG_0/1 -> Reshape1/1
  Reshape1/1 -> First_order_filter_MIMO1/2
  tau_d/1 -> num. derivative/1(x[n])
  CG_0/1 -> num. derivative/2(CG_0), num. derivative2/2(CG_0)
  tau/1 -> num. derivative2/1(x[n])
  reset/1 -> First_order_filter_MIMO1/3, num. derivative/3(reset), num. derivative2/3(reset)
  Product1/1 -> I_out/1

== system Copy_of_minimal_rcu_full/Ipol/joint_ipol_5th_traj_scaling/Subsystem/Cartesian_ipol1/translation/nan_chk5 ==
  in : Inport
  Add : Sum
  Compare To Zero : simulink/Logic and Bit Operations/Compare To Zero  relop===  OutDataTypeStr=uint8  ZeroCross=off
  Compare To Zero1 : simulink/Logic and Bit Operations/Compare To Zero  relop=>  OutDataTypeStr=uint8  ZeroCross=off
  Constant2 : Constant  Value=sample_time_model
  Discrete Derivative2 : simulink/Discrete/Discrete Derivative  gainval=1.0  ICPrevScaledInput=0.0  InputProcessing=Inherited  OutMin=[]  OutMax=[]  OutDataType=sfix(16)  OutScaling=2^-10  DoSatur=off
  Display1 : Display
  Product1 : Product  RndMeth=Zero
  Relational Operator : RelationalOperator  Operator===  OutDataTypeStr=boolean
  Sum of Elements : Sum  Inputs=+
  Switch : Switch  Criteria=u2 > Threshold
  Unit Delay1 : UnitDelay  SampleTime=-1
  in_checked : Outport
  wires:
  Compare To Zero1/1 -> Display1/1, Switch/2
  Sum of Elements/1 -> Compare To Zero1/1
  Compare To Zero/1 -> Sum of Elements/1
  Relational Operator/1 -> Compare To Zero/1
  in/1 -> Relational Operator/1, Relational Operator/2, Switch/3
  Switch/1 -> in_checked/1, Discrete Derivative2/1, Add/1
  Constant2/1 -> Product1/2
  Discrete Derivative2/1 -> Product1/1
  Product1/1 -> Add/2
  Add/1 -> Unit Delay1/1
  Unit Delay1/1 -> Switch/1

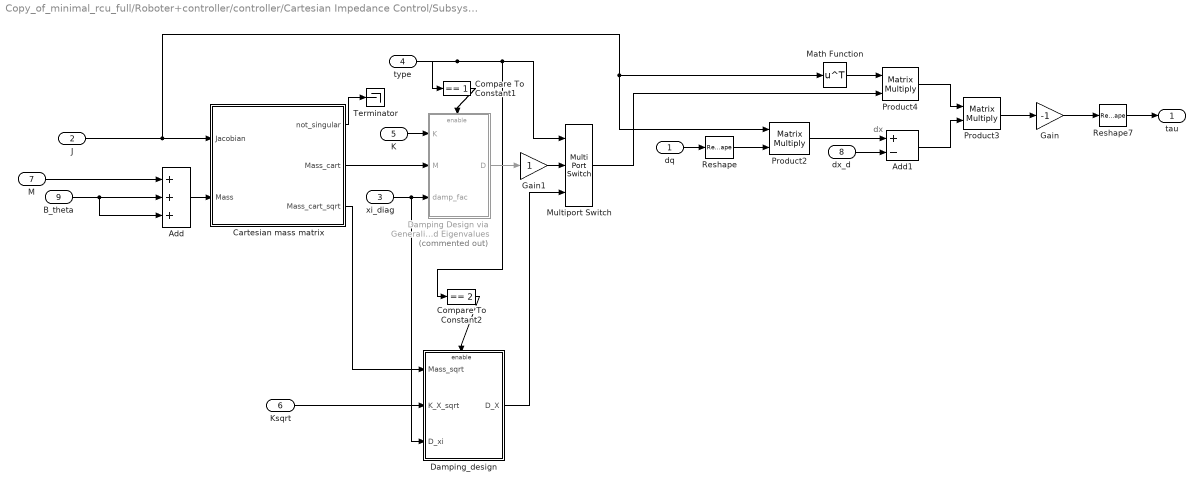
== system Copy_of_minimal_rcu_full/Roboter+controller/controller/Cartesian Impedance Control/Subsystem/Cartesian Compliance Control/Cartesian Damping ==
  note: dx
  dq : Inport
  J : Inport  Port=2
  xi_diag : Inport  Port=3
  type : Inport  Port=4
  K : Inport  Port=5
  Ksqrt : Inport  Port=6
  M : Inport  Port=7
  dx_d : Inport  Port=8
  B_theta : Inport  Port=9
  Add : Sum  Inputs=+++
  Add1 : Sum  Inputs=+-
  Cartesian mass matrix : Subsystem
  Compare To Constant1 : simulink/Logic and Bit Operations/Compare To Constant  relop===  const=1  OutDataTypeStr=uint8  ZeroCross=off
  Compare To Constant2 : simulink/Logic and Bit Operations/Compare To Constant  relop===  const=2  OutDataTypeStr=uint8  ZeroCross=off
  Damping Design via Generalized Eigenvalues : Subsystem  Commented=on  TreatAsAtomicUnit=on
  Damping_design : Subsystem  TreatAsAtomicUnit=on
  Gain : Gain  Gain=-1
  Gain1 : Gain
  Math Function : Math  Operator=transpose  SaturateOnIntegerOverflow=on
  Multiport Switch : MultiPortSwitch  Inputs=2
  Product2 : Product  Multiplication=Matrix(*)  RndMeth=Zero
  Product3 : Product  Multiplication=Matrix(*)  RndMeth=Zero
  Product4 : Product  Multiplication=Matrix(*)  RndMeth=Zero
  Reshape : Reshape  OutputDimensionality=Column vector (2-D)
  Reshape7 : Reshape  OutputDimensions=[7,6]
  Terminator : Terminator
  tau : Outport
  wires:
  xi_diag/1 -> Damping Design via Generalized Eigenvalues/3(damp_fac), Damping_design/3(D_xi)
  Math Function/1 -> Product4/1
  J/1 -> Math Function/1, Product2/1, Cartesian mass matrix/1(Jacobian)
  dq/1 -> Reshape/1
  Gain/1 -> Reshape7/1
  Cartesian mass matrix/2(Mass_cart) -> Damping Design via Generalized Eigenvalues/2(M)
  K/1 -> Damping Design via Generalized Eigenvalues/1(K)
  Add/1 -> Cartesian mass matrix/2(Mass)
  M/1 -> Add/1
  Ksqrt/1 -> Damping_design/2(K_X_sqrt)
  Compare To Constant2/1 -> Damping_design/Enable
  Compare To Constant1/1 -> Damping Design via Generalized Eigenvalues/Enable
  type/1 -> Compare To Constant1/1, Compare To Constant2/1, Multiport Switch/1
  Damping Design via Generalized Eigenvalues/1(D) -> Gain1/1
  Damping_design/1(D_X) -> Multiport Switch/3
  Cartesian mass matrix/3(Mass_cart_sqrt) -> Damping_design/1(Mass_sqrt)
  Multiport Switch/1 -> Product4/2
  Product4/1 -> Product3/1
  Product2/1 -> Add1/1
  Add1/1 -> Product3/2
  Product3/1 -> Gain/1
  dx_d/1 -> Add1/2
  B_theta/1 -> Add/2, Add/3
  Reshape7/1 -> tau/1
  Gain1/1 -> Multiport Switch/2
  Cartesian mass matrix/1(not_singular) -> Terminator/1
  Reshape/1 -> Product2/2
